simulink model "laba5_QPSK3"  (Simulink 7.5)
settings: Solver=ode45  StartTime=0.0  StopTime=10.0  RelTol=1e-3
undefined symbols (not defined in the file): get
libraries: commsink2 x3, commutil2 x2, commdigbbndpm3 x2, commchan3 x1, commrandsrc2 x1
settings Model: Creator=Lenovo  LastModifiedBy=Lenovo

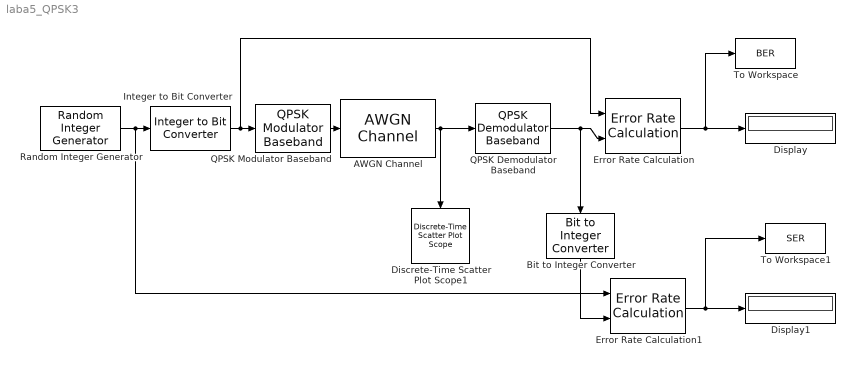
== system laba5_QPSK3 ==
  AWGN Channel : commchan3/AWGN Channel  SystemSampleTime=-1  seed=67  noiseMode="Signal to noise ratio  (Eb/No)"  EbNodB=30  EsNodB=10  SNRdB=10  bitsPerSym=1  Ps=1  Tsym=1  variance=1
  Bit to Integer Converter : commutil2/Bit to Integer Converter  nbits=3  bitOrder=MSB first  signedOutputValues=Unsigned  outDtype=Inherit via internal rule  outDtypeSigned=Inherit via internal rule
  Discrete-Time Scatter Plot Scope1 : commsink2/Discrete-Time Scatter Plot Scope  Tag=ScatterPlot  SystemSampleTime=-1  sampPerSymb=1  offsetEye=0  numTraces=40  numNewFrames=10  LineMarkers=.  LineColors=b  fading=on  render=on  AxisGrid=on  xMin=-3.3  xMax=3.315  yMin=-3.3  yMax=3.315  inphaseLabel=In-phase Amplitude  quadratureLabel=Quadrature Amplitude  openScopeAtSimStart=on  FrameNumber=off  FigPos=get(0,'defaultfigureposition');  figTitle=Scatter Plot  numLinesMax=8  block_type_=scatter
  Display : Display
      settings: Tag=Display
  Display1 : Display
      settings: Tag=Display
  Error Rate Calculation : commsink2/Error Rate Calculation  N=0  st_delay=0  cp_mode=Entire frame  subframe=[]  PMode=Port  WsName=ErrorVec  RsMode2=off  stop=off  numErr=100  maxBits=1e6
  Error Rate Calculation1 : commsink2/Error Rate Calculation  N=0  st_delay=0  cp_mode=Entire frame  subframe=[]  PMode=Port  WsName=ErrorVec  RsMode2=off  stop=off  numErr=100  maxBits=1e6
  Integer to Bit Converter : commutil2/Integer to Bit Converter  nbits=3  signedInputValues=Unsigned  bitOrder=MSB first  outDtype=Inherit via internal rule
  QPSK Demodulator Baseband : commdigbbndpm3/QPSK Demodulator Baseband  DialogController=commDDGCreate  DialogControllerArgs=DataTag0  Ph=pi/4  Dec=Binary  OutType=Integer  DecType=Hard decision  VarSource=Dialog  Variance=1  outDtype1=Inherit via internal rule  outDtype2=Inherit via internal rule  derotateFactorWordLen=16
  QPSK Modulator Baseband : commdigbbndpm3/QPSK Modulator Baseband  DialogController=commDDGCreate  DialogControllerArgs=DataTag1  SystemSampleTime=-1  InType=Integer  Enc=Binary  Ph=pi/4  outDtype=double  outWordLen=16  outUDDataType=sfix(16)  outFracLenMode=Best precision  outFracLen=15
  Random Integer Generator : commrandsrc2/Random Integer Generator  SystemSampleTime=-1  mul=8  seed=37  Ts=1/(38400/544*200)  frameBased=on  sampPerFrame=1  orient=off  outDataType=double
  To Workspace : ToWorkspace  VariableName=BER  SampleTime=-1  SaveFormat=Structure
  To Workspace1 : ToWorkspace  VariableName=SER  SampleTime=-1  SaveFormat=Structure
  wires:
  AWGN Channel/1 -> Discrete-Time Scatter Plot Scope1/1, QPSK Demodulator Baseband/1
  QPSK Demodulator Baseband/1 -> Bit to Integer Converter/1, Error Rate Calculation/2
  Error Rate Calculation/1 -> Display/1, To Workspace/1
  Bit to Integer Converter/1 -> Error Rate Calculation1/2
  Error Rate Calculation1/1 -> Display1/1, To Workspace1/1
  Random Integer Generator/1 -> Integer to Bit Converter/1, Error Rate Calculation1/1
  QPSK Modulator Baseband/1 -> AWGN Channel/1
  Integer to Bit Converter/1 -> QPSK Modulator Baseband/1, Error Rate Calculation/1
